simulink model "BrushedDC"  (R2024b)
settings: Solver=ode45  StartTime=0.0  StopTime=10  FixedStep=0.0001  RelTol=1e-3
model workspace (MAT data in the model file):
  F = 1.65e-07
  J = 2e-07
  K_t = 0.0015
  L = 0.00024
  R = 2.1
libraries: slpidlib x1
settings Model: Creator=Daniil  LastModifiedBy=Daniil
settings DataIOCC: ExternalInput=TestSignals.getElement('torque_load_nm'),TestSignals.getElement('speed_set_hz')  LoadExternalInput=on
settings OptimizationCC: DefaultUnderspecifiedDataType=single
settings RTWCC: BuildConfiguration=Debug  GPUComputeCapability=3.5

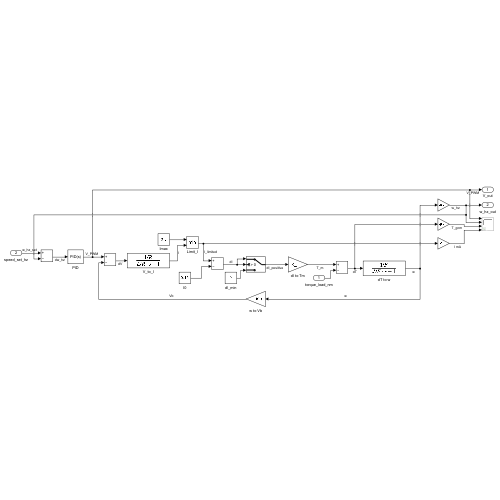
[thumbnail: Simulink's stored preview of the top-level diagram]
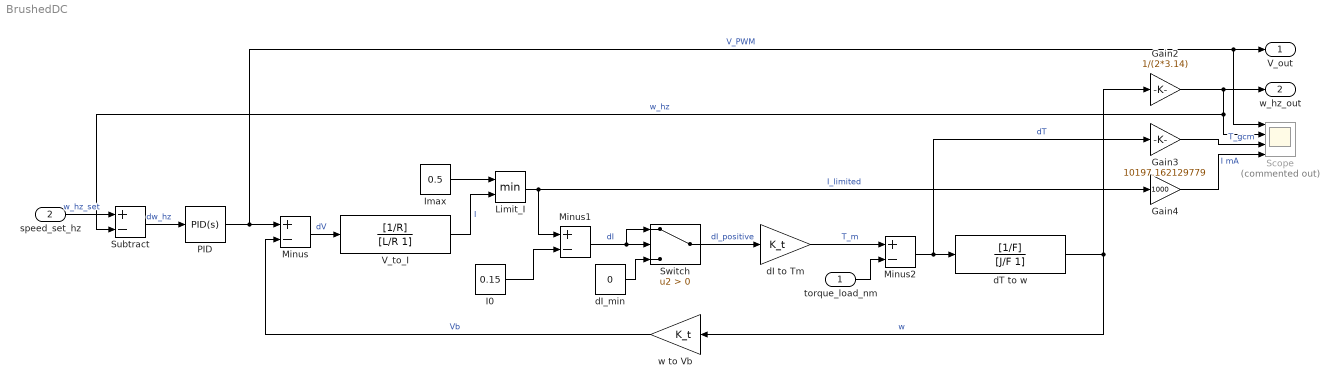
== system BrushedDC ==
  torque_load_nm : Inport  PortDimensions=1
  speed_set_hz : Inport  Port=2  PortDimensions=1
  Gain2 : Gain  Gain=1/(2*3.14)
  Gain3 : Gain  Gain=10197.162129779
  Gain4 : Gain  Gain=1000
  I0 : Constant  Value=0.15
  Imax : Constant  Value=0.5
  Limit_I : MinMax  Inputs=2
  Minus : Sum  Inputs=+-
  Minus1 : Sum  Inputs=+-
  Minus2 : Sum  Inputs=+-
  PID : slpidlib/PID Controller  Controller=PID  Form=Parallel  TimeDomain=Continuous-time  UseExternalTs=off  SampleTime=-1  IntegratorMethod=Forward Euler  FilterMethod=Forward Euler  ControllerParametersSource=internal  P=0.03  I=0.05  UseKiTs=off  D=0  UseExternalDerivativeSource=off  N=100  UseFilter=on  TunerSelectOption=Transfer Function Based (PID Tuner App)  InitialConditionSource=internal  InitialConditionForIntegrator=0  InitialConditionForFilter=0  DifferentiatorICPrevScaledInput=0  ExternalReset=none  TrackingMode=off  Kt=1  LimitOutput=off  SatLimitsSource=internal  UpperSaturationLimit=inf  LowerSaturationLimit=-inf  LinearizeAsGain=on  AntiWindupMode=none  Kb=1  LimitIntegrator=off  UpperIntegratorSaturationLimit=inf  LowerIntegratorSaturationLimit=-inf  POutMin=[]  POutMax=[]  IOutMin=[]  IOutMax=[]  DOutMin=[]  DOutMax=[]  NOutMin=[]  NOutMax=[]  SumOutMin=[]  SumOutMax=[]  SaturationOutMin=[]  SaturationOutMax=[]  PParamMin=[]  PParamMax=[]  IParamMin=[]  IParamMax=[]  DParamMin=[]  DParamMax=[]  NParamMin=[]  NParamMax=[]  KbParamMin=[]  KbParamMax=[]  KtParamMin=[]  KtParamMax=[]  KbOutMin=[]  KbOutMax=[]  KtOutMin=[]  KtOutMax=[]  IntegratorOutMin=[]  IntegratorOutMax=[]  FilterOutMin=[]  FilterOutMax=[]  SumI1OutMin=[]  SumI1OutMax=[]  SumI2OutMin=[]  SumI2OutMax=[]  SumI3OutMin=[]  SumI3OutMax=[]  SumI4OutMin=[]  SumI4OutMax=[]  SumDOutMin=[]  SumDOutMax=[]  DifferentiatorOutMin=[]  DifferentiatorOutMax=[]  FilterDiffOutCoefMin=[]  FilterDiffOutCoefMax=[]  ReciprocalOutMin=[]  ReciprocalOutMax=[]  SumDenOutMin=[]  SumDenOutMax=[]  SumNumOutMin=[]  SumNumOutMax=[]  DivideOutMin=[]  DivideOutMax=[]  UdiffTsProdOutMin=[]  UdiffTsProdOutMax=[]  NTsProdOutMin=[]  NTsProdOutMax=[]  UintegralTsProdOutMin=[]  UintegralTsProdOutMax=[]  UngainTsProdOutMin=[]  UngainTsProdOutMax=[]  ClampingZeroOutDataTypeStr=Inherit: Inherit via back propagation  ClampingZeroOutMin=[]  ClampingZeroOutMax=[]  FilterDenConstantOutDataTypeStr=Inherit: Inherit via back propagation  FilterDenConstantOutMin=[]  FilterDenConstantOutMax=[]  PCopyOutDataTypeStr=Inherit: Inherit via back propagation  PCopyOutMin=[]  PCopyOutMax=[]  NCopyOutDataTypeStr=Inherit: Inherit via back propagation  NCopyOutMin=[]  NCopyOutMax=[]  IntegratorContinuousStateAttributes=''  IntegratorStateMustResolveToSignalObject=off  IntegratorRTWStateStorageClass=Auto  FilterContinuousStateAttributes=''  FilterStateMustResolveToSignalObject=off  FilterRTWStateStorageClass=Auto  ParallelPVariant=InternalParameters  IdealPVariant=Disabled  IVariant=InternalParameters  DVariant=InternalParameters  IntegratorVariant=Continuous  SatVariant=Disabled  AWVariant=Passthrough  PCopyVariant=Disabled  TRVariant=Disabled  FdbkBlocksVariant=Forward  IdealPFdbkVariant=Disabled  SatFdbkVariant=Disabled  DerivativeFilterVariant=ContFilter  NVariant=InternalParameters  NCopyVariant=Disabled  FilterICVariant=InternalICsFilter  IntegratorICVariant=InternalICs  ExternalResetVariant=Disabled  TRSumVariant=Passthrough  SumFdbkVariant=Disabled  SumVariant=Sum_PID  TsampFilterVariant=InternalTs  TsampNgainVariant=Passthrough  TsampIntegralVariant=Disabled_SignalSpec  ExternalSaturationOutDataTypeStr=Inherit: Same as second input  DerivativeSourceVariant=ErrorSignal  PreIntVariant=InternalPreInt
  Scope : Scope  Commented=on  NumInputPorts=4
  Subtract : Sum  Inputs=+-
  Switch : Switch  Criteria=u2 > Threshold  SaturateOnIntegerOverflow=off  InputSameDT=off
  V_to_I : TransferFcn  Numerator=[1/R]  Denominator=[L/R 1]
  dI to Tm : Gain  Gain=K_t
  dI_min : Constant  Value=0
  dT to w : TransferFcn  Numerator=[1/F]  Denominator=[J/F 1]
  w to Vb : Gain  Gain=K_t
  V_out : Outport
  w_hz_out : Outport  Port=2
  wires:
  I0/1 -> Minus1/2
  Minus1/1 -> Switch/1, Switch/2  "dI"
  Minus/1 -> V_to_I/1  "dV"
  dI to Tm/1 -> Minus2/1  "T_m"
  Minus2/1 -> Gain3/1, dT to w/1  "dT"
  dT to w/1 -> w to Vb/1, Gain2/1  "w"
  w to Vb/1 -> Minus/2  "Vb"
  dI_min/1 -> Switch/3
  Gain4/1 -> Scope/4  "I mA"
  Gain3/1 -> Scope/3  "T_gcm"
  Gain2/1 -> Scope/2, Subtract/2, w_hz_out/1  "w_hz"
  PID/1 -> Scope/1, V_out/1, Minus/1  "V_PWM"
  speed_set_hz/1 -> Subtract/1  "w_hz_set"
  Subtract/1 -> PID/1  "dw_hz"
  Switch/1 -> dI to Tm/1  "dI_positive"
  Limit_I/1 -> Gain4/1, Minus1/1  "I_limited"
  torque_load_nm/1 -> Minus2/2
  Imax/1 -> Limit_I/1
  V_to_I/1 -> Limit_I/2  "I"
